simulink model "Active_Cell_BalancingBuck_Boost_12CeLL_KSB"  (R2023b)
settings: Solver=VariableStepAuto  StartTime=0.0  StopTime=300  MaxStep=1e-4  MinStep=1e-5  RelTol=1e-3
undefined symbols (not defined in the file): Ion, Lithium
libraries: spsIdealSwitchLib x26, spsSeriesRLCBranchLib x26, spsDiodeLib x24, spsBatteryLib x12, spsDCVoltageSourceLib x1, spsPWMGenerator2LevelLib x1, sps_lib x1
settings Model: Creator=home  LastModifiedBy=Kumar Bhaweshnu
settings OptimizationCC: ReuseModelBlockBuffer=off

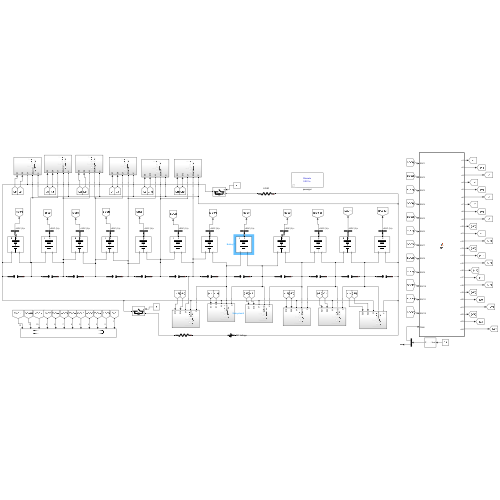
[thumbnail: Simulink's stored preview of the top-level diagram]
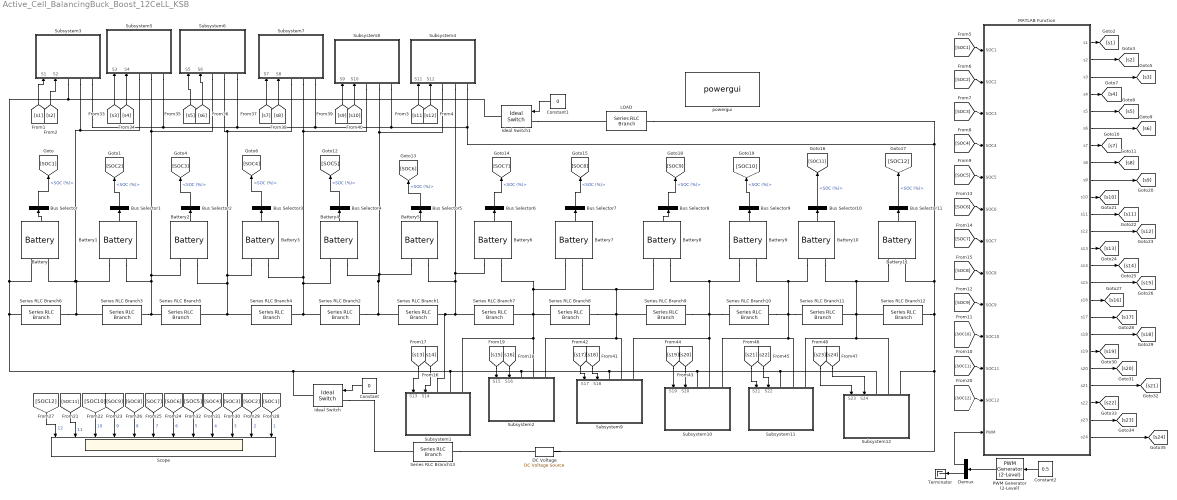
== system Active_Cell_BalancingBuck_Boost_12CeLL_KSB ==
  Battery : spsBatteryLib/Battery  BatType=Lithium-Ion  ShowTempParam=off  ThermalPreset=no  ShowAgeParam=off  NomV=3.7  NomQ=5.4  SOC=45  Batt_Tr=30  PresetModel=on  MaxQ=5.4  MinV=2.775  FullV=4.3068  Dis_rate=2.3478  R=0.0068519  Normal_OP=4.8835  expZone="[3.9974      0.2653]"  current=[6.5 13 32.5]  Units=Time  Tci=20  NomT=20  T2=-30  MaxQ2=4.8  FullV2=7.1  Normal_OP2=5.655  expZone2="[6.58           1]"  Rca=0.6  ti=2000  Dp=0  Neq0=0  Tsim=1e6  Ta1=25  Qeol=5.4*0.9  Reol=0.013333*1.2  Char_age=[2.3478, 3]  Dis_age=[2.3478, 10]  N1=1500  N2=10500  N3=1000  N4=1400  Ta2=45  N5=950
  Battery1 : spsBatteryLib/Battery  BatType=Lithium-Ion  ShowTempParam=off  ThermalPreset=no  ShowAgeParam=off  NomV=3.7  NomQ=5.4  SOC=50  Batt_Tr=30  PresetModel=on  MaxQ=5.4  MinV=2.775  FullV=4.3068  Dis_rate=2.3478  R=0.0068519  Normal_OP=4.8835  expZone="[3.9974      0.2653]"  current=[6.5 13 32.5]  Units=Time  Tci=20  NomT=20  T2=-30  MaxQ2=4.8  FullV2=7.1  Normal_OP2=5.655  expZone2="[6.58           1]"  Rca=0.6  ti=2000  Dp=0  Neq0=0  Tsim=1e6  Ta1=25  Qeol=5.4*0.9  Reol=0.013333*1.2  Char_age=[2.3478, 3]  Dis_age=[2.3478, 10]  N1=1500  N2=10500  N3=1000  N4=1400  Ta2=45  N5=950
  Battery10 : spsBatteryLib/Battery  BatType=Lithium-Ion  ShowTempParam=off  ThermalPreset=no  ShowAgeParam=off  NomV=3.7  NomQ=5.4  SOC=46.3  Batt_Tr=30  PresetModel=on  MaxQ=5.4  MinV=2.775  FullV=4.3068  Dis_rate=2.3478  R=0.0068519  Normal_OP=4.8835  expZone="[3.9974      0.2653]"  current=[6.5 13 32.5]  Units=Time  Tci=20  NomT=20  T2=-30  MaxQ2=4.8  FullV2=7.1  Normal_OP2=5.655  expZone2="[6.58           1]"  Rca=0.6  ti=2000  Dp=0  Neq0=0  Tsim=1e6  Ta1=25  Qeol=5.4*0.9  Reol=0.013333*1.2  Char_age=[2.3478, 3]  Dis_age=[2.3478, 10]  N1=1500  N2=10500  N3=1000  N4=1400  Ta2=45  N5=950
  Battery11 : spsBatteryLib/Battery  BatType=Lithium-Ion  ShowTempParam=off  ThermalPreset=no  ShowAgeParam=off  NomV=3.7  NomQ=5.4  SOC=48.2  Batt_Tr=30  PresetModel=on  MaxQ=5.4  MinV=2.775  FullV=4.3068  Dis_rate=2.3478  R=0.0068519  Normal_OP=4.8835  expZone="[3.9974      0.2653]"  current=[6.5 13 32.5]  Units=Time  Tci=20  NomT=20  T2=-30  MaxQ2=4.8  FullV2=7.1  Normal_OP2=5.655  expZone2="[6.58           1]"  Rca=0.6  ti=2000  Dp=0  Neq0=0  Tsim=1e6  Ta1=25  Qeol=5.4*0.9  Reol=0.013333*1.2  Char_age=[2.3478, 3]  Dis_age=[2.3478, 10]  N1=1500  N2=10500  N3=1000  N4=1400  Ta2=45  N5=950
  Battery2 : spsBatteryLib/Battery  BatType=Lithium-Ion  ShowTempParam=off  ThermalPreset=no  ShowAgeParam=off  NomV=3.7  NomQ=5.4  SOC=49.8  Batt_Tr=30  PresetModel=on  MaxQ=5.4  MinV=2.775  FullV=4.3068  Dis_rate=2.3478  R=0.0068519  Normal_OP=4.8835  expZone="[3.9974      0.2653]"  current=[6.5 13 32.5]  Units=Time  Tci=20  NomT=20  T2=-30  MaxQ2=4.8  FullV2=7.1  Normal_OP2=5.655  expZone2="[6.58           1]"  Rca=0.6  ti=2000  Dp=0  Neq0=0  Tsim=1e6  Ta1=25  Qeol=5.4*0.9  Reol=0.013333*1.2  Char_age=[2.3478, 3]  Dis_age=[2.3478, 10]  N1=1500  N2=10500  N3=1000  N4=1400  Ta2=45  N5=950
  Battery3 : spsBatteryLib/Battery  BatType=Lithium-Ion  ShowTempParam=off  ThermalPreset=no  ShowAgeParam=off  NomV=3.7  NomQ=5.4  SOC=48  Batt_Tr=30  PresetModel=on  MaxQ=5.4  MinV=2.775  FullV=4.3068  Dis_rate=2.3478  R=0.0068519  Normal_OP=4.8835  expZone="[3.9974      0.2653]"  current=[6.5 13 32.5]  Units=Time  Tci=20  NomT=20  T2=-30  MaxQ2=4.8  FullV2=7.1  Normal_OP2=5.655  expZone2="[6.58           1]"  Rca=0.6  ti=2000  Dp=0  Neq0=0  Tsim=1e6  Ta1=25  Qeol=5.4*0.9  Reol=0.013333*1.2  Char_age=[2.3478, 3]  Dis_age=[2.3478, 10]  N1=1500  N2=10500  N3=1000  N4=1400  Ta2=45  N5=950
  Battery4 : spsBatteryLib/Battery  BatType=Lithium-Ion  ShowTempParam=off  ThermalPreset=no  ShowAgeParam=off  NomV=3.7  NomQ=5.4  SOC=48.1  Batt_Tr=30  PresetModel=on  MaxQ=5.4  MinV=2.775  FullV=4.3068  Dis_rate=2.3478  R=0.0068519  Normal_OP=4.8835  expZone="[3.9974      0.2653]"  current=[6.5 13 32.5]  Units=Time  Tci=20  NomT=20  T2=-30  MaxQ2=4.8  FullV2=7.1  Normal_OP2=5.655  expZone2="[6.58           1]"  Rca=0.6  ti=2000  Dp=0  Neq0=0  Tsim=1e6  Ta1=25  Qeol=5.4*0.9  Reol=0.013333*1.2  Char_age=[2.3478, 3]  Dis_age=[2.3478, 10]  N1=1500  N2=10500  N3=1000  N4=1400  Ta2=45  N5=950
  Battery5 : spsBatteryLib/Battery  BatType=Lithium-Ion  ShowTempParam=off  ThermalPreset=no  ShowAgeParam=off  NomV=3.7  NomQ=5.4  SOC=48.3  Batt_Tr=30  PresetModel=on  MaxQ=5.4  MinV=2.775  FullV=4.3068  Dis_rate=2.3478  R=0.0068519  Normal_OP=4.8835  expZone="[3.9974      0.2653]"  current=[6.5 13 32.5]  Units=Time  Tci=20  NomT=20  T2=-30  MaxQ2=4.8  FullV2=7.1  Normal_OP2=5.655  expZone2="[6.58           1]"  Rca=0.6  ti=2000  Dp=0  Neq0=0  Tsim=1e6  Ta1=25  Qeol=5.4*0.9  Reol=0.013333*1.2  Char_age=[2.3478, 3]  Dis_age=[2.3478, 10]  N1=1500  N2=10500  N3=1000  N4=1400  Ta2=45  N5=950
  Battery6 : spsBatteryLib/Battery  BatType=Lithium-Ion  ShowTempParam=off  ThermalPreset=no  ShowAgeParam=off  NomV=3.7  NomQ=5.4  SOC=46.8  Batt_Tr=30  PresetModel=on  MaxQ=5.4  MinV=2.775  FullV=4.3068  Dis_rate=2.3478  R=0.0068519  Normal_OP=4.8835  expZone="[3.9974      0.2653]"  current=[6.5 13 32.5]  Units=Time  Tci=20  NomT=20  T2=-30  MaxQ2=4.8  FullV2=7.1  Normal_OP2=5.655  expZone2="[6.58           1]"  Rca=0.6  ti=2000  Dp=0  Neq0=0  Tsim=1e6  Ta1=25  Qeol=5.4*0.9  Reol=0.013333*1.2  Char_age=[2.3478, 3]  Dis_age=[2.3478, 10]  N1=1500  N2=10500  N3=1000  N4=1400  Ta2=45  N5=950
  Battery7 : spsBatteryLib/Battery  BatType=Lithium-Ion  ShowTempParam=off  ThermalPreset=no  ShowAgeParam=off  NomV=3.7  NomQ=5.4  SOC=48.7  Batt_Tr=30  PresetModel=on  MaxQ=5.4  MinV=2.775  FullV=4.3068  Dis_rate=2.3478  R=0.0068519  Normal_OP=4.8835  expZone="[3.9974      0.2653]"  current=[6.5 13 32.5]  Units=Time  Tci=20  NomT=20  T2=-30  MaxQ2=4.8  FullV2=7.1  Normal_OP2=5.655  expZone2="[6.58           1]"  Rca=0.6  ti=2000  Dp=0  Neq0=0  Tsim=1e6  Ta1=25  Qeol=5.4*0.9  Reol=0.013333*1.2  Char_age=[2.3478, 3]  Dis_age=[2.3478, 10]  N1=1500  N2=10500  N3=1000  N4=1400  Ta2=45  N5=950
  Battery8 : spsBatteryLib/Battery  BatType=Lithium-Ion  ShowTempParam=off  ThermalPreset=no  ShowAgeParam=off  NomV=3.7  NomQ=5.4  SOC=49.4  Batt_Tr=30  PresetModel=on  MaxQ=5.4  MinV=2.775  FullV=4.3068  Dis_rate=2.3478  R=0.0068519  Normal_OP=4.8835  expZone="[3.9974      0.2653]"  current=[6.5 13 32.5]  Units=Time  Tci=20  NomT=20  T2=-30  MaxQ2=4.8  FullV2=7.1  Normal_OP2=5.655  expZone2="[6.58           1]"  Rca=0.6  ti=2000  Dp=0  Neq0=0  Tsim=1e6  Ta1=25  Qeol=5.4*0.9  Reol=0.013333*1.2  Char_age=[2.3478, 3]  Dis_age=[2.3478, 10]  N1=1500  N2=10500  N3=1000  N4=1400  Ta2=45  N5=950
  Battery9 : spsBatteryLib/Battery  BatType=Lithium-Ion  ShowTempParam=off  ThermalPreset=no  ShowAgeParam=off  NomV=3.7  NomQ=5.4  SOC=48.9  Batt_Tr=30  PresetModel=on  MaxQ=5.4  MinV=2.775  FullV=4.3068  Dis_rate=2.3478  R=0.0068519  Normal_OP=4.8835  expZone="[3.9974      0.2653]"  current=[6.5 13 32.5]  Units=Time  Tci=20  NomT=20  T2=-30  MaxQ2=4.8  FullV2=7.1  Normal_OP2=5.655  expZone2="[6.58           1]"  Rca=0.6  ti=2000  Dp=0  Neq0=0  Tsim=1e6  Ta1=25  Qeol=5.4*0.9  Reol=0.013333*1.2  Char_age=[2.3478, 3]  Dis_age=[2.3478, 10]  N1=1500  N2=10500  N3=1000  N4=1400  Ta2=45  N5=950
  Bus Selector{,1..11} (12 alike) : BusSelector  OutputSignals=SOC (%)
  Constant : Constant  Value=0
  Constant1 : Constant  Value=0
  Constant2 : Constant  Value=0.5
  DC Voltage : spsDCVoltageSourceLib/DC Voltage Source  Amplitude=48  Measurements=None
  Demux : Demux  Outputs=2
  Ideal Switch : spsIdealSwitchLib/Ideal Switch  Ron=0.001  Lon=0  IC=0  Rs=1e5  Cs=inf  Measurements=off
  Ideal Switch1 : spsIdealSwitchLib/Ideal Switch  Ron=0.001  Lon=0  IC=0  Rs=1e5  Cs=inf  Measurements=off
  LOAD : spsSeriesRLCBranchLib/Series RLC Branch  LConnTagsString=__new0  RConnTagsString=__new0  BranchType=R  Resistance=1  Inductance=1e-3  SetiL0=off  InitialCurrent=0  Capacitance=1e-6  Setx0=off  InitialVoltage=0  Measurements=None
  MATLAB Function : MATLAB Function  TreatAsAtomicUnit=on
  PWM Generator (2-Level) : spsPWMGenerator2LevelLib/PWM Generator (2-Level)  ModulatorType=Single-phase half-bridge (2 pulses)  ModulatorMode=Unsynchronized  Fc=100  Pc=0  nF=27  MinMax="[ -1  1 ]"  SamplingTechnique=Natural  ModulatingSignals=off  m=0.8  Freq=60  Phase=0  Ts=0  ShowCarrierOutport=off
  Scope : Scope  NumInputPorts=12
  Series RLC Branch{1..12} (12 alike) : spsSeriesRLCBranchLib/Series RLC Branch  LConnTagsString=__new0  RConnTagsString=__new0  BranchType=C  Resistance=1  Inductance=1e-3  SetiL0=off  InitialCurrent=0  Capacitance=1e-6  Setx0=off  InitialVoltage=0  Measurements=None
  Series RLC Branch13 : spsSeriesRLCBranchLib/Series RLC Branch  LConnTagsString=__new0  RConnTagsString=__new0  BranchType=R  Resistance=0.01  Inductance=1e-3  SetiL0=off  InitialCurrent=0  Capacitance=1e-6  Setx0=off  InitialVoltage=0  Measurements=None
  Subsystem1 : Subsystem
  Subsystem10 : Subsystem
  Subsystem11 : Subsystem
  Subsystem12 : Subsystem
  Subsystem2 : Subsystem
  Subsystem3 : Subsystem
  Subsystem4 : Subsystem
  Subsystem5 : Subsystem
  Subsystem6 : Subsystem
  Subsystem7 : Subsystem
  Subsystem8 : Subsystem
  Subsystem9 : Subsystem
  Terminator : Terminator
  powergui : sps_lib/powergui  Priority=1  SimulationMode=Discrete  SampleTime=1000e-6  frequency=60  Iterations=50  frequencyindice=0  Pbase=100e6  ErrMax=1e-4  UnitsV=kV  UnitsW=MW  buscounter=0  FunctionMessages=off  echomessages=off  EnableUseOfTLC=off  CurrentSourceSwitches=off  DisableSnubberDevices=off  DisableRonSwitches=off  DisableVfSwitches=off  DisplayEquations=off  AutomaticDiscreteSolvers=off  SolverType=Tustin/Backward Euler (TBE)  Interpol=off  ExternalGateDelay=off  methode=off  Ts=100  x0status=blocks  SPID=on  SwTol=0  HookPort=off  NonlinearTolerance=1e-4  nMaxIteration=100  ContinueOnMaxIteration=off  RestoreLinks=warning  ResistiveCurrentMeasurement=off  Frange=[0:2:500]  Ylog=off  Xlog=on  ShowGrid=off  save=off  variable=ZData  structure=0  ZoomFFT=off  StartTime=0.0  cycles=1  DisplayStyle=1  fundamental=60  FreqAxis=off  MaxFrequency=1000  frequencyindicesteady=1  RmsSteady=1  display=off
  wires:
  [SOC6] -> Scope/7  "6"
  [SOC2] -> Scope/11  "2"
  [SOC11] -> Scope/2  "11"
  [SOC9] -> Scope/4  "9"
  [SOC3] -> Scope/10  "3"
  [SOC7] -> Scope/6  "7"
  [SOC8] -> Scope/5  "8"
  [SOC10] -> Scope/3  "10"
  MATLAB Function/11(s11) -> [s11]
  MATLAB Function/23(s23) -> [s23]
  MATLAB Function/20(s20) -> [s20]
  [s13] -> Subsystem1/1(S13)
  [s14] -> Subsystem1/2(S14)
  MATLAB Function/24(s24) -> [s24]
  [s18] -> Subsystem9/2(S18)
  MATLAB Function/1(s1) -> [s1]
  [SOC4] -> MATLAB Function/4(SOC4)
  [SOC10] -> MATLAB Function/10(SOC10)
  Bus Selector9/1 -> [SOC10]  "<SOC (%)>"
  MATLAB Function/6(s6) -> [s6]
  MATLAB Function/7(s7) -> [s7]
  Bus Selector11/1 -> [SOC12]  "<SOC (%)>"
  Bus Selector6/1 -> [SOC7]  "<SOC (%)>"
  Demux/1 -> MATLAB Function/13(PWM)
  [SOC7] -> MATLAB Function/7(SOC7)
  MATLAB Function/8(s8) -> [s8]
  Bus Selector4/1 -> [SOC5]  "<SOC (%)>"
  [s12] -> Subsystem4/2(S12)
  MATLAB Function/18(s18) -> [s18]
  [SOC8] -> MATLAB Function/8(SOC8)
  PWM Generator (2-Level)/1 -> Demux/1
  Battery11/1 -> Bus Selector11/1
  [s1] -> Subsystem3/1(S1)
  Battery6/1 -> Bus Selector6/1
  Bus Selector5/1 -> [SOC6]  "<SOC (%)>"
  Bus Selector1/1 -> [SOC2]  "<SOC (%)>"
  Bus Selector/1 -> [SOC1]  "<SOC (%)>"
  [SOC4] -> Scope/9  "4"
  Battery5/1 -> Bus Selector5/1
  MATLAB Function/2(s2) -> [s2]
  MATLAB Function/5(s5) -> [s5]
  Constant2/1 -> PWM Generator (2-Level)/1
  [s2] -> Subsystem3/2(S2)
  [SOC2] -> MATLAB Function/2(SOC2)
  [SOC6] -> MATLAB Function/6(SOC6)
  [SOC1] -> Scope/12  "1"
  [SOC12] -> Scope/1  "12"
  [s17] -> Subsystem9/1(S17)
  MATLAB Function/3(s3) -> [s3]
  Bus Selector3/1 -> [SOC4]  "<SOC (%)>"
  [SOC1] -> MATLAB Function/1(SOC1)
  MATLAB Function/4(s4) -> [s4]
  Battery9/1 -> Bus Selector9/1
  Battery3/1 -> Bus Selector3/1
  Bus Selector8/1 -> [SOC9]  "<SOC (%)>"
  Bus Selector2/1 -> [SOC3]  "<SOC (%)>"
  [s11] -> Subsystem4/1(S11)
  [SOC12] -> MATLAB Function/12(SOC12)
  Battery4/1 -> Bus Selector4/1
  [s20] -> Subsystem10/2(S20)
  Battery1/1 -> Bus Selector1/1
  Bus Selector7/1 -> [SOC8]  "<SOC (%)>"
  [SOC3] -> MATLAB Function/3(SOC3)
  Bus Selector10/1 -> [SOC11]  "<SOC (%)>"
  [s23] -> Subsystem12/1(S23)
  [s24] -> Subsystem12/2(S24)
  [s15] -> Subsystem2/1(S15)
  Battery8/1 -> Bus Selector8/1
  [SOC11] -> MATLAB Function/11(SOC11)
  [s10] -> Subsystem8/2(S10)
  MATLAB Function/16(s16) -> [s16]
  [s3] -> Subsystem5/1(S3)
  [s5] -> Subsystem6/1(S5)
  MATLAB Function/22(s22) -> [s22]
  MATLAB Function/14(s14) -> [s14]
  Battery10/1 -> Bus Selector10/1
  [s7] -> Subsystem7/1(S7)
  [SOC9] -> MATLAB Function/9(SOC9)
  [s8] -> Subsystem7/2(S8)
  [s19] -> Subsystem10/1(S19)
  MATLAB Function/12(s12) -> [s12]
  [s21] -> Subsystem11/1(S21)
  [SOC5] -> MATLAB Function/5(SOC5)
  [s22] -> Subsystem11/2(S22)
  MATLAB Function/19(s19) -> [s19]
  MATLAB Function/15(s15) -> [s15]
  MATLAB Function/21(s21) -> [s21]
  MATLAB Function/17(s17) -> [s17]
  MATLAB Function/13(s13) -> [s13]
  [s9] -> Subsystem8/1(S9)
  MATLAB Function/10(s10) -> [s10]
  [s16] -> Subsystem2/2(S16)
  MATLAB Function/9(s9) -> [s9]
  Battery/1 -> Bus Selector/1
  [s4] -> Subsystem5/2(S4)
  Battery2/1 -> Bus Selector2/1
  [SOC5] -> Scope/8  "5"
  [s6] -> Subsystem6/2(S6)
  Battery7/1 -> Bus Selector7/1
  Demux/2 -> Terminator/1
  Constant/1 -> Ideal Switch/1
  Constant1/1 -> Ideal Switch1/1
  connections:
  Battery5/LConn1 -- Battery4/LConn2 -- Series RLC Branch2/LConn1 -- Series RLC Branch1/RConn1 -- Subsystem4/LConn1 -- Subsystem8/LConn2
  Subsystem6/LConn2 -- Subsystem7/LConn1 -- Series RLC Branch4/RConn1 -- Series RLC Branch5/LConn1 -- Battery2/LConn2 -- Battery3/LConn1
  Battery5/LConn2 -- Battery6/LConn1 -- Subsystem4/LConn2 -- Subsystem1/LConn1 -- Series RLC Branch1/LConn1 -- Series RLC Branch7/RConn1
  Battery11/LConn2 -- LOAD/LConn1 -- Subsystem3/LConn3 -- Subsystem5/LConn3 -- Subsystem6/LConn3 -- Subsystem7/LConn3 -- Subsystem8/LConn3 -- Subsystem4/LConn3 -- DC Voltage/LConn1 -- Subsystem12/LConn3 -- Series RLC Branch12/LConn1
  Subsystem3/LConn2 -- Battery1/LConn1 -- Series RLC Branch3/RConn1 -- Series RLC Branch6/LConn1 -- Battery/LConn2 -- Subsystem5/LConn1
  Series RLC Branch10/RConn1 -- Subsystem9/LConn3 -- Subsystem10/LConn2 -- Series RLC Branch9/LConn1 -- Battery8/LConn2 -- Battery9/LConn1
  Series RLC Branch7/LConn1 -- Subsystem1/LConn3 -- Subsystem2/LConn2 -- Series RLC Branch8/RConn1 -- Battery6/LConn2 -- Battery7/LConn1
  Subsystem10/LConn1 -- Subsystem12/LConn1 -- Subsystem11/LConn1 -- Subsystem2/LConn1 -- Ideal Switch1/RConn1 -- Subsystem3/LConn1 -- Battery/LConn1 -- Series RLC Branch6/RConn1 -- Ideal Switch/RConn1 -- Subsystem1/LConn2 -- Subsystem9/LConn1
  Subsystem12/LConn2 -- Subsystem11/LConn3 -- Series RLC Branch11/LConn1 -- Battery10/LConn2 -- Battery11/LConn1 -- Series RLC Branch12/RConn1
  Battery1/LConn2 -- Subsystem6/LConn1 -- Subsystem5/LConn2 -- Battery2/LConn1 -- Series RLC Branch5/RConn1 -- Series RLC Branch3/LConn1
  Subsystem9/LConn2 -- Subsystem2/LConn3 -- Series RLC Branch8/LConn1 -- Battery8/LConn1 -- Battery7/LConn2 -- Series RLC Branch9/RConn1
  Series RLC Branch11/RConn1 -- Subsystem10/LConn3 -- Subsystem11/LConn2 -- Series RLC Branch10/LConn1 -- Battery9/LConn2 -- Battery10/LConn1
  Subsystem7/LConn2 -- Subsystem8/LConn1 -- Battery4/LConn1 -- Series RLC Branch2/RConn1 -- Series RLC Branch4/LConn1 -- Battery3/LConn2
  Series RLC Branch13/LConn1 -- DC Voltage/RConn1
  Ideal Switch/LConn1 -- Series RLC Branch13/RConn1
  Ideal Switch1/LConn1 -- LOAD/RConn1

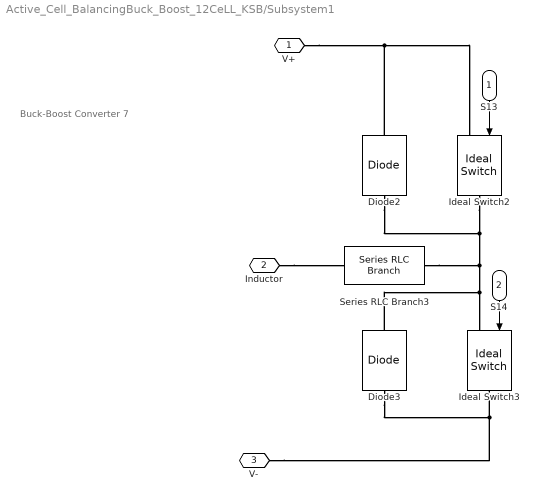
== system Active_Cell_BalancingBuck_Boost_12CeLL_KSB/Subsystem1 ==
  note: Buck-Boost Converter 7
  S13 : Inport
  S14 : Inport  Port=2
  Diode2 : spsDiodeLib/Diode  Ron=0.001  Lon=0  Vf=0.8  IC=0  UseSnubber=0  Rs=500  Cs=250e-9  Measurements=off
  Diode3 : spsDiodeLib/Diode  Ron=0.001  Lon=0  Vf=0.8  IC=0  UseSnubber=0  Rs=500  Cs=250e-9  Measurements=off
  Ideal Switch2 : spsIdealSwitchLib/Ideal Switch  Ron=0.001  Lon=0  IC=0  Rs=1e5  Cs=inf  Measurements=off
  Ideal Switch3 : spsIdealSwitchLib/Ideal Switch  Ron=0.001  Lon=0  IC=0  Rs=1e5  Cs=inf  Measurements=off
  Series RLC Branch3 : spsSeriesRLCBranchLib/Series RLC Branch  LConnTagsString=__new0  RConnTagsString=__new0  BranchType=L  Resistance=1  Inductance=1e-3  SetiL0=off  InitialCurrent=0  Capacitance=1e-6  Setx0=off  InitialVoltage=0  Measurements=None
  V+ : PMIOPort  Side=Left
  Inductor : PMIOPort  Port=2  Side=Left
  V- : PMIOPort  Port=3  Side=Left
  wires:
  S13/1 -> Ideal Switch2/1
  S14/1 -> Ideal Switch3/1
  connections:
  Inductor/RConn1 -- Series RLC Branch3/LConn1
  Diode2/LConn1 -- Series RLC Branch3/RConn1 -- Diode3/RConn1 -- Ideal Switch3/LConn1 -- Ideal Switch2/RConn1
  Diode2/RConn1 -- Ideal Switch2/LConn1 -- V+/RConn1
  Diode3/LConn1 -- Ideal Switch3/RConn1 -- V-/RConn1

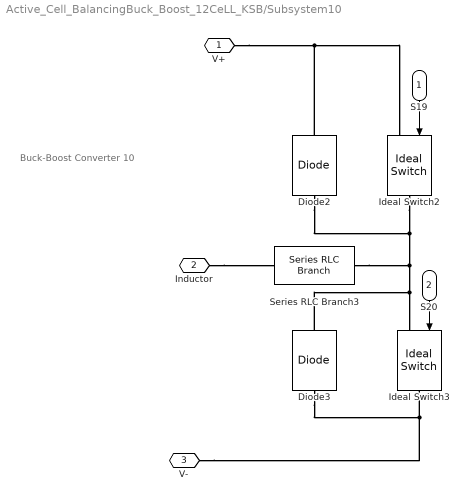
== system Active_Cell_BalancingBuck_Boost_12CeLL_KSB/Subsystem10 ==
  note: Buck-Boost Converter 10
  S19 : Inport
  S20 : Inport  Port=2
  Diode2 : spsDiodeLib/Diode  Ron=0.001  Lon=0  Vf=0.8  IC=0  UseSnubber=0  Rs=500  Cs=250e-9  Measurements=off
  Diode3 : spsDiodeLib/Diode  Ron=0.001  Lon=0  Vf=0.8  IC=0  UseSnubber=0  Rs=500  Cs=250e-9  Measurements=off
  Ideal Switch2 : spsIdealSwitchLib/Ideal Switch  Ron=0.001  Lon=0  IC=0  Rs=1e5  Cs=inf  Measurements=off
  Ideal Switch3 : spsIdealSwitchLib/Ideal Switch  Ron=0.001  Lon=0  IC=0  Rs=1e5  Cs=inf  Measurements=off
  Series RLC Branch3 : spsSeriesRLCBranchLib/Series RLC Branch  LConnTagsString=__new0  RConnTagsString=__new0  BranchType=L  Resistance=1  Inductance=1e-3  SetiL0=off  InitialCurrent=0  Capacitance=1e-6  Setx0=off  InitialVoltage=0  Measurements=None
  V+ : PMIOPort  Side=Left
  Inductor : PMIOPort  Port=2  Side=Left
  V- : PMIOPort  Port=3  Side=Left
  wires:
  S20/1 -> Ideal Switch3/1
  S19/1 -> Ideal Switch2/1
  connections:
  V-/RConn1 -- Ideal Switch3/RConn1 -- Diode3/LConn1
  V+/RConn1 -- Ideal Switch2/LConn1 -- Diode2/RConn1
  Ideal Switch2/RConn1 -- Ideal Switch3/LConn1 -- Diode3/RConn1 -- Series RLC Branch3/RConn1 -- Diode2/LConn1
  Inductor/RConn1 -- Series RLC Branch3/LConn1

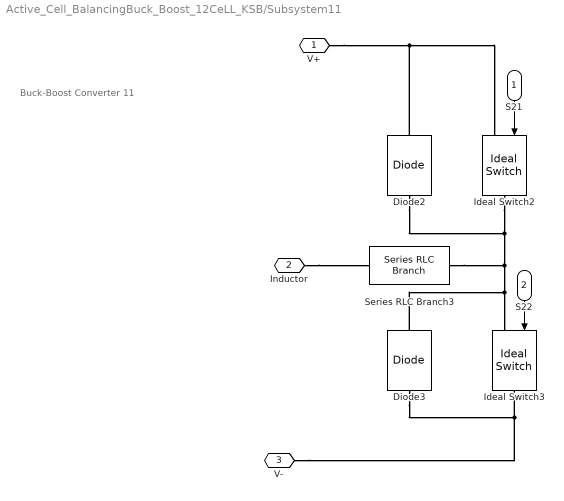
== system Active_Cell_BalancingBuck_Boost_12CeLL_KSB/Subsystem11 ==
  note: Buck-Boost Converter 11
  S21 : Inport
  S22 : Inport  Port=2
  Diode2 : spsDiodeLib/Diode  Ron=0.001  Lon=0  Vf=0.8  IC=0  UseSnubber=0  Rs=500  Cs=250e-9  Measurements=off
  Diode3 : spsDiodeLib/Diode  Ron=0.001  Lon=0  Vf=0.8  IC=0  UseSnubber=0  Rs=500  Cs=250e-9  Measurements=off
  Ideal Switch2 : spsIdealSwitchLib/Ideal Switch  Ron=0.001  Lon=0  IC=0  Rs=1e5  Cs=inf  Measurements=off
  Ideal Switch3 : spsIdealSwitchLib/Ideal Switch  Ron=0.001  Lon=0  IC=0  Rs=1e5  Cs=inf  Measurements=off
  Series RLC Branch3 : spsSeriesRLCBranchLib/Series RLC Branch  LConnTagsString=__new0  RConnTagsString=__new0  BranchType=L  Resistance=1  Inductance=1e-3  SetiL0=off  InitialCurrent=0  Capacitance=1e-6  Setx0=off  InitialVoltage=0  Measurements=None
  V+ : PMIOPort  Side=Left
  Inductor : PMIOPort  Port=2  Side=Left
  V- : PMIOPort  Port=3  Side=Left
  wires:
  S21/1 -> Ideal Switch2/1
  S22/1 -> Ideal Switch3/1
  connections:
  Inductor/RConn1 -- Series RLC Branch3/LConn1
  Diode2/LConn1 -- Series RLC Branch3/RConn1 -- Diode3/RConn1 -- Ideal Switch3/LConn1 -- Ideal Switch2/RConn1
  Diode2/RConn1 -- Ideal Switch2/LConn1 -- V+/RConn1
  Diode3/LConn1 -- Ideal Switch3/RConn1 -- V-/RConn1

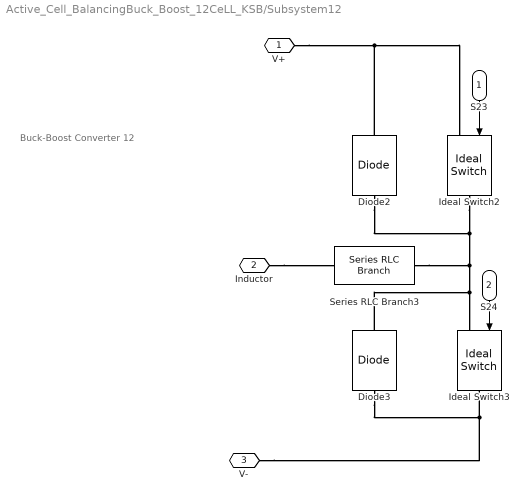
== system Active_Cell_BalancingBuck_Boost_12CeLL_KSB/Subsystem12 ==
  note: Buck-Boost Converter 12
  S23 : Inport
  S24 : Inport  Port=2
  Diode2 : spsDiodeLib/Diode  Ron=0.001  Lon=0  Vf=0.8  IC=0  UseSnubber=0  Rs=500  Cs=250e-9  Measurements=off
  Diode3 : spsDiodeLib/Diode  Ron=0.001  Lon=0  Vf=0.8  IC=0  UseSnubber=0  Rs=500  Cs=250e-9  Measurements=off
  Ideal Switch2 : spsIdealSwitchLib/Ideal Switch  Ron=0.001  Lon=0  IC=0  Rs=1e5  Cs=inf  Measurements=off
  Ideal Switch3 : spsIdealSwitchLib/Ideal Switch  Ron=0.001  Lon=0  IC=0  Rs=1e5  Cs=inf  Measurements=off
  Series RLC Branch3 : spsSeriesRLCBranchLib/Series RLC Branch  LConnTagsString=__new0  RConnTagsString=__new0  BranchType=L  Resistance=1  Inductance=1e-3  SetiL0=off  InitialCurrent=0  Capacitance=1e-6  Setx0=off  InitialVoltage=0  Measurements=None
  V+ : PMIOPort  Side=Left
  Inductor : PMIOPort  Port=2  Side=Left
  V- : PMIOPort  Port=3  Side=Left
  wires:
  S24/1 -> Ideal Switch3/1
  S23/1 -> Ideal Switch2/1
  connections:
  V-/RConn1 -- Ideal Switch3/RConn1 -- Diode3/LConn1
  V+/RConn1 -- Ideal Switch2/LConn1 -- Diode2/RConn1
  Ideal Switch2/RConn1 -- Ideal Switch3/LConn1 -- Diode3/RConn1 -- Series RLC Branch3/RConn1 -- Diode2/LConn1
  Inductor/RConn1 -- Series RLC Branch3/LConn1

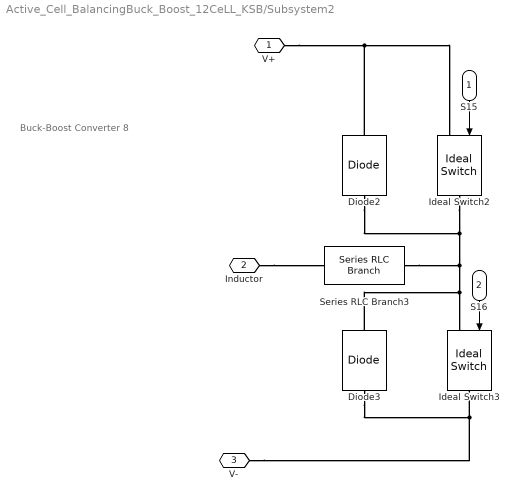
== system Active_Cell_BalancingBuck_Boost_12CeLL_KSB/Subsystem2 ==
  note: Buck-Boost Converter 8
  S15 : Inport
  S16 : Inport  Port=2
  Diode2 : spsDiodeLib/Diode  Ron=0.001  Lon=0  Vf=0.8  IC=0  UseSnubber=0  Rs=500  Cs=250e-9  Measurements=off
  Diode3 : spsDiodeLib/Diode  Ron=0.001  Lon=0  Vf=0.8  IC=0  UseSnubber=0  Rs=500  Cs=250e-9  Measurements=off
  Ideal Switch2 : spsIdealSwitchLib/Ideal Switch  Ron=0.001  Lon=0  IC=0  Rs=1e5  Cs=inf  Measurements=off
  Ideal Switch3 : spsIdealSwitchLib/Ideal Switch  Ron=0.001  Lon=0  IC=0  Rs=1e5  Cs=inf  Measurements=off
  Series RLC Branch3 : spsSeriesRLCBranchLib/Series RLC Branch  LConnTagsString=__new0  RConnTagsString=__new0  BranchType=L  Resistance=1  Inductance=1e-3  SetiL0=off  InitialCurrent=0  Capacitance=1e-6  Setx0=off  InitialVoltage=0  Measurements=None
  V+ : PMIOPort  Side=Left
  Inductor : PMIOPort  Port=2  Side=Left
  V- : PMIOPort  Port=3  Side=Left
  wires:
  S16/1 -> Ideal Switch3/1
  S15/1 -> Ideal Switch2/1
  connections:
  V-/RConn1 -- Ideal Switch3/RConn1 -- Diode3/LConn1
  V+/RConn1 -- Ideal Switch2/LConn1 -- Diode2/RConn1
  Ideal Switch2/RConn1 -- Ideal Switch3/LConn1 -- Diode3/RConn1 -- Series RLC Branch3/RConn1 -- Diode2/LConn1
  Inductor/RConn1 -- Series RLC Branch3/LConn1

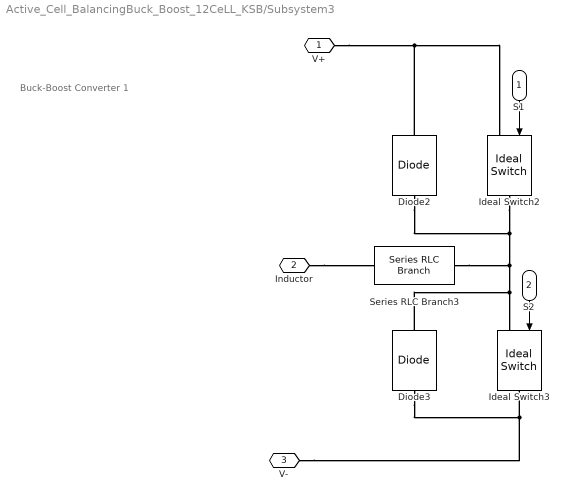
== system Active_Cell_BalancingBuck_Boost_12CeLL_KSB/Subsystem3 ==
  note: Buck-Boost Converter 1
  S1 : Inport
  S2 : Inport  Port=2
  Diode2 : spsDiodeLib/Diode  Ron=0.001  Lon=0  Vf=0.8  IC=0  UseSnubber=0  Rs=500  Cs=250e-9  Measurements=off
  Diode3 : spsDiodeLib/Diode  Ron=0.001  Lon=0  Vf=0.8  IC=0  UseSnubber=0  Rs=500  Cs=250e-9  Measurements=off
  Ideal Switch2 : spsIdealSwitchLib/Ideal Switch  Ron=0.001  Lon=0  IC=0  Rs=1e5  Cs=inf  Measurements=off
  Ideal Switch3 : spsIdealSwitchLib/Ideal Switch  Ron=0.001  Lon=0  IC=0  Rs=1e5  Cs=inf  Measurements=off
  Series RLC Branch3 : spsSeriesRLCBranchLib/Series RLC Branch  LConnTagsString=__new0  RConnTagsString=__new0  BranchType=L  Resistance=1  Inductance=1e-3  SetiL0=off  InitialCurrent=0  Capacitance=1e-6  Setx0=off  InitialVoltage=0  Measurements=None
  V+ : PMIOPort  Side=Left
  Inductor : PMIOPort  Port=2  Side=Left
  V- : PMIOPort  Port=3  Side=Left
  wires:
  S1/1 -> Ideal Switch2/1
  S2/1 -> Ideal Switch3/1
  connections:
  Inductor/RConn1 -- Series RLC Branch3/LConn1
  Diode2/LConn1 -- Series RLC Branch3/RConn1 -- Diode3/RConn1 -- Ideal Switch3/LConn1 -- Ideal Switch2/RConn1
  Diode2/RConn1 -- Ideal Switch2/LConn1 -- V+/RConn1
  Diode3/LConn1 -- Ideal Switch3/RConn1 -- V-/RConn1

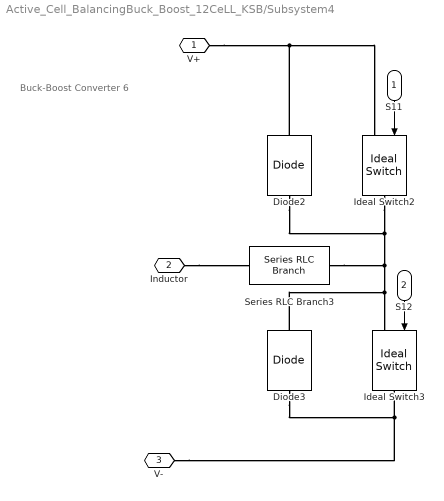
== system Active_Cell_BalancingBuck_Boost_12CeLL_KSB/Subsystem4 ==
  note: Buck-Boost Converter 6
  S11 : Inport
  S12 : Inport  Port=2
  Diode2 : spsDiodeLib/Diode  Ron=0.001  Lon=0  Vf=0.8  IC=0  UseSnubber=0  Rs=500  Cs=250e-9  Measurements=off
  Diode3 : spsDiodeLib/Diode  Ron=0.001  Lon=0  Vf=0.8  IC=0  UseSnubber=0  Rs=500  Cs=250e-9  Measurements=off
  Ideal Switch2 : spsIdealSwitchLib/Ideal Switch  Ron=0.001  Lon=0  IC=0  Rs=1e5  Cs=inf  Measurements=off
  Ideal Switch3 : spsIdealSwitchLib/Ideal Switch  Ron=0.001  Lon=0  IC=0  Rs=1e5  Cs=inf  Measurements=off
  Series RLC Branch3 : spsSeriesRLCBranchLib/Series RLC Branch  LConnTagsString=__new0  RConnTagsString=__new0  BranchType=L  Resistance=1  Inductance=1e-3  SetiL0=off  InitialCurrent=0  Capacitance=1e-6  Setx0=off  InitialVoltage=0  Measurements=None
  V+ : PMIOPort  Side=Left
  Inductor : PMIOPort  Port=2  Side=Left
  V- : PMIOPort  Port=3  Side=Left
  wires:
  S11/1 -> Ideal Switch2/1
  S12/1 -> Ideal Switch3/1
  connections:
  Inductor/RConn1 -- Series RLC Branch3/LConn1
  Diode2/LConn1 -- Series RLC Branch3/RConn1 -- Diode3/RConn1 -- Ideal Switch3/LConn1 -- Ideal Switch2/RConn1
  Diode2/RConn1 -- Ideal Switch2/LConn1 -- V+/RConn1
  Diode3/LConn1 -- Ideal Switch3/RConn1 -- V-/RConn1

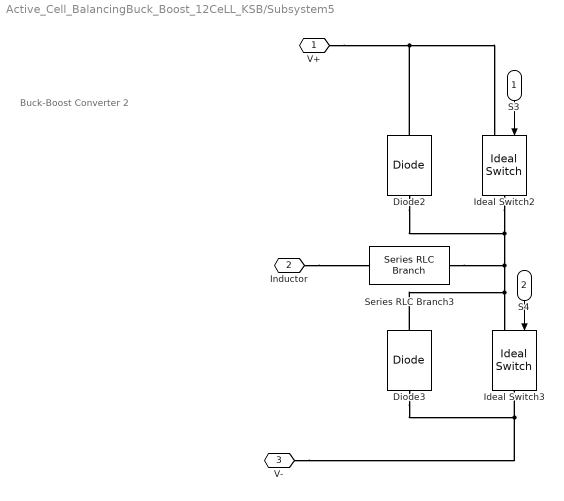
== system Active_Cell_BalancingBuck_Boost_12CeLL_KSB/Subsystem5 ==
  note: Buck-Boost Converter 2
  S3 : Inport
  S4 : Inport  Port=2
  Diode2 : spsDiodeLib/Diode  Ron=0.001  Lon=0  Vf=0.8  IC=0  UseSnubber=0  Rs=500  Cs=250e-9  Measurements=off
  Diode3 : spsDiodeLib/Diode  Ron=0.001  Lon=0  Vf=0.8  IC=0  UseSnubber=0  Rs=500  Cs=250e-9  Measurements=off
  Ideal Switch2 : spsIdealSwitchLib/Ideal Switch  Ron=0.001  Lon=0  IC=0  Rs=1e5  Cs=inf  Measurements=off
  Ideal Switch3 : spsIdealSwitchLib/Ideal Switch  Ron=0.001  Lon=0  IC=0  Rs=1e5  Cs=inf  Measurements=off
  Series RLC Branch3 : spsSeriesRLCBranchLib/Series RLC Branch  LConnTagsString=__new0  RConnTagsString=__new0  BranchType=L  Resistance=1  Inductance=1e-3  SetiL0=off  InitialCurrent=0  Capacitance=1e-6  Setx0=off  InitialVoltage=0  Measurements=None
  V+ : PMIOPort  Side=Left
  Inductor : PMIOPort  Port=2  Side=Left
  V- : PMIOPort  Port=3  Side=Left
  wires:
  S3/1 -> Ideal Switch2/1
  S4/1 -> Ideal Switch3/1
  connections:
  Inductor/RConn1 -- Series RLC Branch3/LConn1
  Diode2/LConn1 -- Series RLC Branch3/RConn1 -- Diode3/RConn1 -- Ideal Switch3/LConn1 -- Ideal Switch2/RConn1
  Diode2/RConn1 -- Ideal Switch2/LConn1 -- V+/RConn1
  Diode3/LConn1 -- Ideal Switch3/RConn1 -- V-/RConn1

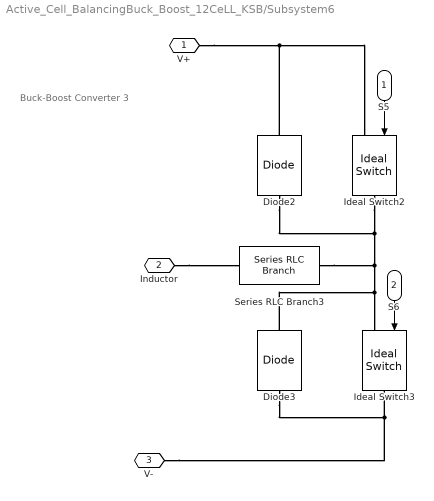
== system Active_Cell_BalancingBuck_Boost_12CeLL_KSB/Subsystem6 ==
  note: Buck-Boost Converter 3
  S5 : Inport
  S6 : Inport  Port=2
  Diode2 : spsDiodeLib/Diode  Ron=0.001  Lon=0  Vf=0.8  IC=0  UseSnubber=0  Rs=500  Cs=250e-9  Measurements=off
  Diode3 : spsDiodeLib/Diode  Ron=0.001  Lon=0  Vf=0.8  IC=0  UseSnubber=0  Rs=500  Cs=250e-9  Measurements=off
  Ideal Switch2 : spsIdealSwitchLib/Ideal Switch  Ron=0.001  Lon=0  IC=0  Rs=1e5  Cs=inf  Measurements=off
  Ideal Switch3 : spsIdealSwitchLib/Ideal Switch  Ron=0.001  Lon=0  IC=0  Rs=1e5  Cs=inf  Measurements=off
  Series RLC Branch3 : spsSeriesRLCBranchLib/Series RLC Branch  LConnTagsString=__new0  RConnTagsString=__new0  BranchType=L  Resistance=1  Inductance=1e-3  SetiL0=off  InitialCurrent=0  Capacitance=1e-6  Setx0=off  InitialVoltage=0  Measurements=None
  V+ : PMIOPort  Side=Left
  Inductor : PMIOPort  Port=2  Side=Left
  V- : PMIOPort  Port=3  Side=Left
  wires:
  S5/1 -> Ideal Switch2/1
  S6/1 -> Ideal Switch3/1
  connections:
  Inductor/RConn1 -- Series RLC Branch3/LConn1
  Diode2/LConn1 -- Series RLC Branch3/RConn1 -- Diode3/RConn1 -- Ideal Switch3/LConn1 -- Ideal Switch2/RConn1
  Diode2/RConn1 -- Ideal Switch2/LConn1 -- V+/RConn1
  Diode3/LConn1 -- Ideal Switch3/RConn1 -- V-/RConn1

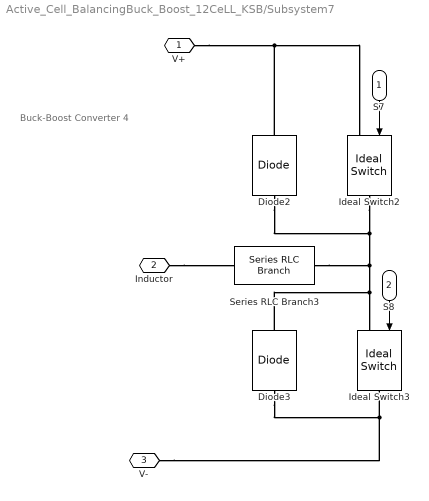
== system Active_Cell_BalancingBuck_Boost_12CeLL_KSB/Subsystem7 ==
  note: Buck-Boost Converter 4
  S7 : Inport
  S8 : Inport  Port=2
  Diode2 : spsDiodeLib/Diode  Ron=0.001  Lon=0  Vf=0.8  IC=0  UseSnubber=0  Rs=500  Cs=250e-9  Measurements=off
  Diode3 : spsDiodeLib/Diode  Ron=0.001  Lon=0  Vf=0.8  IC=0  UseSnubber=0  Rs=500  Cs=250e-9  Measurements=off
  Ideal Switch2 : spsIdealSwitchLib/Ideal Switch  Ron=0.001  Lon=0  IC=0  Rs=1e5  Cs=inf  Measurements=off
  Ideal Switch3 : spsIdealSwitchLib/Ideal Switch  Ron=0.001  Lon=0  IC=0  Rs=1e5  Cs=inf  Measurements=off
  Series RLC Branch3 : spsSeriesRLCBranchLib/Series RLC Branch  LConnTagsString=__new0  RConnTagsString=__new0  BranchType=L  Resistance=1  Inductance=1e-3  SetiL0=off  InitialCurrent=0  Capacitance=1e-6  Setx0=off  InitialVoltage=0  Measurements=None
  V+ : PMIOPort  Side=Left
  Inductor : PMIOPort  Port=2  Side=Left
  V- : PMIOPort  Port=3  Side=Left
  wires:
  S7/1 -> Ideal Switch2/1
  S8/1 -> Ideal Switch3/1
  connections:
  Inductor/RConn1 -- Series RLC Branch3/LConn1
  Diode2/LConn1 -- Series RLC Branch3/RConn1 -- Diode3/RConn1 -- Ideal Switch3/LConn1 -- Ideal Switch2/RConn1
  Diode2/RConn1 -- Ideal Switch2/LConn1 -- V+/RConn1
  Diode3/LConn1 -- Ideal Switch3/RConn1 -- V-/RConn1

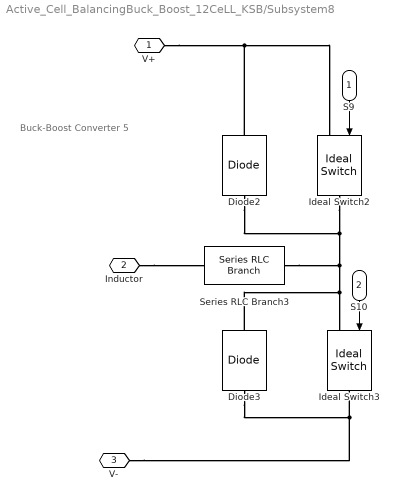
== system Active_Cell_BalancingBuck_Boost_12CeLL_KSB/Subsystem8 ==
  note: Buck-Boost Converter 5
  S9 : Inport
  S10 : Inport  Port=2
  Diode2 : spsDiodeLib/Diode  Ron=0.001  Lon=0  Vf=0.8  IC=0  UseSnubber=0  Rs=500  Cs=250e-9  Measurements=off
  Diode3 : spsDiodeLib/Diode  Ron=0.001  Lon=0  Vf=0.8  IC=0  UseSnubber=0  Rs=500  Cs=250e-9  Measurements=off
  Ideal Switch2 : spsIdealSwitchLib/Ideal Switch  Ron=0.001  Lon=0  IC=0  Rs=1e5  Cs=inf  Measurements=off
  Ideal Switch3 : spsIdealSwitchLib/Ideal Switch  Ron=0.001  Lon=0  IC=0  Rs=1e5  Cs=inf  Measurements=off
  Series RLC Branch3 : spsSeriesRLCBranchLib/Series RLC Branch  LConnTagsString=__new0  RConnTagsString=__new0  BranchType=L  Resistance=1  Inductance=1e-3  SetiL0=off  InitialCurrent=0  Capacitance=1e-6  Setx0=off  InitialVoltage=0  Measurements=None
  V+ : PMIOPort  Side=Left
  Inductor : PMIOPort  Port=2  Side=Left
  V- : PMIOPort  Port=3  Side=Left
  wires:
  S9/1 -> Ideal Switch2/1
  S10/1 -> Ideal Switch3/1
  connections:
  Inductor/RConn1 -- Series RLC Branch3/LConn1
  Diode2/LConn1 -- Series RLC Branch3/RConn1 -- Diode3/RConn1 -- Ideal Switch3/LConn1 -- Ideal Switch2/RConn1
  Diode2/RConn1 -- Ideal Switch2/LConn1 -- V+/RConn1
  Diode3/LConn1 -- Ideal Switch3/RConn1 -- V-/RConn1

== system Active_Cell_BalancingBuck_Boost_12CeLL_KSB/Subsystem9 ==
  note: Buck-Boost Converter 9
  S17 : Inport
  S18 : Inport  Port=2
  Diode2 : spsDiodeLib/Diode  Ron=0.001  Lon=0  Vf=0.8  IC=0  UseSnubber=0  Rs=500  Cs=250e-9  Measurements=off
  Diode3 : spsDiodeLib/Diode  Ron=0.001  Lon=0  Vf=0.8  IC=0  UseSnubber=0  Rs=500  Cs=250e-9  Measurements=off
  Ideal Switch2 : spsIdealSwitchLib/Ideal Switch  Ron=0.001  Lon=0  IC=0  Rs=1e5  Cs=inf  Measurements=off
  Ideal Switch3 : spsIdealSwitchLib/Ideal Switch  Ron=0.001  Lon=0  IC=0  Rs=1e5  Cs=inf  Measurements=off
  Series RLC Branch3 : spsSeriesRLCBranchLib/Series RLC Branch  LConnTagsString=__new0  RConnTagsString=__new0  BranchType=L  Resistance=1  Inductance=1e-3  SetiL0=off  InitialCurrent=0  Capacitance=1e-6  Setx0=off  InitialVoltage=0  Measurements=None
  V+ : PMIOPort  Side=Left
  Inductor : PMIOPort  Port=2  Side=Left
  V- : PMIOPort  Port=3  Side=Left
  wires:
  S17/1 -> Ideal Switch2/1
  S18/1 -> Ideal Switch3/1
  connections:
  Inductor/RConn1 -- Series RLC Branch3/LConn1
  Diode2/LConn1 -- Series RLC Branch3/RConn1 -- Diode3/RConn1 -- Ideal Switch3/LConn1 -- Ideal Switch2/RConn1
  Diode2/RConn1 -- Ideal Switch2/LConn1 -- V+/RConn1
  Diode3/LConn1 -- Ideal Switch3/RConn1 -- V-/RConn1

== matlab function Active_Cell_BalancingBuck_Boost_12CeLL_KSB/MATLAB Function ==
  data: SOC1 input; s1 output; SOC2 input; SOC3 input; SOC4 input; SOC5 input; SOC6 input; SOC7 input; SOC8 input; SOC9 input; SOC10 input; SOC11 input; SOC12 input; PWM input; s2 output; s3 output; s4 output; s5 output; s6 output; s7 output; s8 output; s9 output; s10 output; s11 output; s12 output; s13 output; s14 output; s15 output; s16 output; s17 output; s18 output; s19 output; s20 output; s21 output; s22 output; s23 output; s24 output
function [s1,s2,s3,s4,s5,s6,s7,s8,s9,s10,s11,s12,s13,s14,s15,s16,s17,s18,s19,s20,s21,s22,s23,s24] = fcn(SOC1,SOC2,SOC3,SOC4,SOC5,SOC6,SOC7,SOC8,SOC9,SOC10,SOC11,SOC12,PWM)

%H = max([SOC1,SOC2,SOC3,SOC4,SOC5,SOC6,SOC7,SOC8,SOC9,SOC10,SOC11,SOC12]);
L = min([SOC1,SOC2,SOC3,SOC4,SOC5,SOC6,SOC7,SOC8,SOC9,SOC10,SOC11,SOC12]);
if L==SOC1
    s1=0;s2=PWM;s3=0;s4=0;s5=0;s6=0;s7=0;s8=0;s9=0;s10=0;s11=0;s12=0;s13=0;s14=0;s15=0;s16=0;s17=0;s18=0;s19=0;s20=0;s21=0;s22=0;s23=0;s24=0;
elseif L==SOC2
    s1=0;s2=0;s3=0;s4=PWM;s5=0;s6=0;s7=0;s8=0;s9=0;s10=0;s11=0;s12=0;s13=0;s14=0;s15=0;s16=0;s17=0;s18=0;s19=0;s20=0;s21=0;s22=0;s23=0;s24=0;
elseif L==SOC3
    s1=0;s2=0;s3=0;s4=0;s5=0;s6=PWM;s7=0;s8=0;s9=0;s10=0;s11=0;s12=0;s13=0;s14=0;s15=0;s16=0;s17=0;s18=0;s19=0;s20=0;s21=0;s22=0;s23=0;s24=0;
elseif L==SOC4
    s1=0;s2=0;s3=0;s4=0;s5=0;s6=0;s7=0;s8=PWM;s9=0;s10=0;s11=0;s12=0;s13=0;s14=0;s15=0;s16=0;s17=0;s18=0;s19=0;s20=0;s21=0;s22=0;s23=0;s24=0;
elseif L==SOC5
    s1=0;s2=0;s3=0;s4=0;s5=0;s6=0;s7=0;s8=0;s9=0;s10=PWM;s11=0;s12=0;s13=0;s14=0;s15=0;s16=0;s17=0;s18=0;s19=0;s20=0;s21=0;s22=0;s23=0;s24=0;
elseif L==SOC6
    s1=0;s2=0;s3=0;s4=0;s5=0;s6=0;s7=0;s8=0;s9=0;s10=0;s11=0;s12=PWM;s13=0;s14=0;s15=0;s16=0;s17=0;s18=0;s19=0;s20=0;s21=0;s22=0;s23=0;s24=0;
elseif L==SOC7
    s1=0;s2=0;s3=0;s4=0;s5=0;s6=0;s7=0;s8=0;s9=0;s10=0;s11=0;s12=0;s13=PWM;s14=0;s15=0;s16=0;s17=0;s18=0;s19=0;s20=0;s21=0;s22=0;s23=0;s24=0;
elseif L==SOC8
    s1=0;s2=0;s3=0;s4=0;s5=0;s6=0;s7=0;s8=0;s9=0;s10=0;s11=0;s12=0;s13=0;s14=0;s15=PWM;s16=0;s17=0;s18=0;s19=0;s20=0;s21=0;s22=0;s23=0;s24=0;
elseif L==SOC9
    s1=0;s2=0;s3=0;s4=0;s5=0;s6=0;s7=0;s8=0;s9=0;s10=0;s11=0;s12=0;s13=0;s14=0;s15=0;s16=0;s17=PWM;s18=0;s19=0;s20=0;s21=0;s22=0;s23=0;s24=0;
elseif L==SOC10
    s1=0;s2=0;s3=0;s4=0;s5=0;s6=0;s7=0;s8=0;s9=0;s10=0;s11=0;s12=0;s13=0;s14=0;s15=0;s16=0;s17=0;s18=0;s19=PWM;s20=0;s21=0;s22=0;s23=0;s24=0;
elseif L==SOC11
    s1=0;s2=0;s3=0;s4=0;s5=0;s6=0;s7=0;s8=0;s9=0;s10=0;s11=0;s12=0;s13=0;s14=0;s15=0;s16=0;s17=0;s18=0;s19=0;s20=0;s21=PWM;s22=0;s23=0;s24=0;
elseif L==SOC12
    s1=0;s2=0;s3=0;s4=0;s5=0;s6=0;s7=0;s8=0;s9=0;s10=0;s11=0;s12=0;s13=0;s14=0;s15=0;s16=0;s17=0;s18=0;s19=0;s20=0;s21=0;s22=0;s23=PWM;s24=0;
else
    s1=0;s2=0;s3=0;s4=0;s5=0;s6=0;s7=0;s8=0;s9=0;s10=0;s11=0;s12=0;s13=0;s14=0;s15=0;s16=0;s17=0;s18=0;s19=0;s20=0;s21=0;s22=0;s23=0;s24=0;

end
end
